simulink model "SPHERE_model"  (R2020a)
settings: Solver=ode4  StartTime=0.0  StopTime=20.0  FixedStep=0.01  RelTol=1e-3
values from neighbouring files (symbols this model uses):
  L = -[ M2*l*(-2*l + R) - 2*J2, 0, -2*M2*l*g ]    [Initial_script.m]    (also in Initial_script_test.m; Initial_script_test2.m)
  M = [ J1 + 2*J2 + M1*R^2 + M2*(2*l^2 - 3*R*l + R^2), -Tv, 2*l*g*M2 ]    [Initial_script.m]    (also in Initial_script_test.m; Initial_script_test2.m)
libraries: simulink x1
settings Model: Creator=Adrian  LastModifiedBy=Adrian

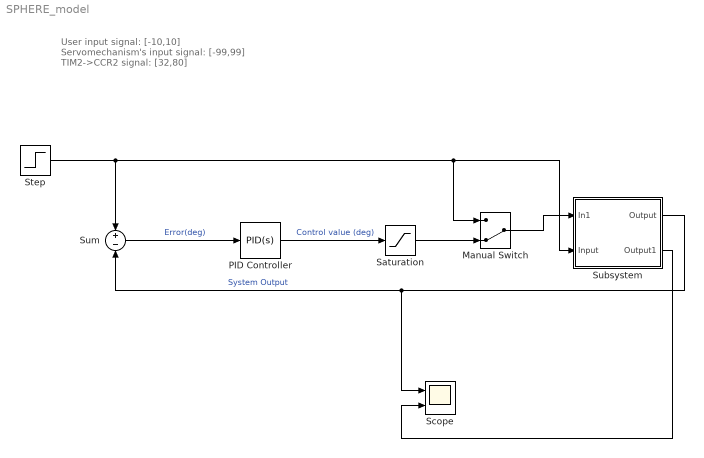
== system SPHERE_model ==
  note: User input signal: [-10,10]
      | Servomechanism's input signal: [-99,99]
      | TIM2->CCR2 signal: [32,80]
  Manual Switch : ManualSwitch  CurrentSetting=0
  PID Controller : simulink/Continuous/PID Controller  Controller=PID  Form=Parallel  TimeDomain=Continuous-time  UseExternalTs=off  SampleTime=-1  IntegratorMethod=Forward Euler  FilterMethod=Forward Euler  ControllerParametersSource=internal  P=1.5  I=0.2  D=0.1  UseFilter=on  N=100  TunerSelectOption=Transfer Function Based (PID Tuner App)  InitialConditionSource=internal  InitialConditionForIntegrator=0  InitialConditionForFilter=0  DifferentiatorICPrevScaledInput=0  ExternalReset=none  TrackingMode=off  Kt=1  LimitOutput=off  UpperSaturationLimit=inf  LowerSaturationLimit=-inf  LinearizeAsGain=on  AntiWindupMode=none  Kb=1  POutMin=[]  POutMax=[]  IOutMin=[]  IOutMax=[]  DOutMin=[]  DOutMax=[]  NOutMin=[]  NOutMax=[]  SumOutMin=[]  SumOutMax=[]  SaturationOutMin=[]  SaturationOutMax=[]  PParamMin=[]  PParamMax=[]  IParamMin=[]  IParamMax=[]  DParamMin=[]  DParamMax=[]  NParamMin=[]  NParamMax=[]  KbParamMin=[]  KbParamMax=[]  KtParamMin=[]  KtParamMax=[]  KbOutMin=[]  KbOutMax=[]  KtOutMin=[]  KtOutMax=[]  IntegratorOutMin=[]  IntegratorOutMax=[]  FilterOutMin=[]  FilterOutMax=[]  SumI1OutMin=[]  SumI1OutMax=[]  SumI2OutMin=[]  SumI2OutMax=[]  SumI3OutMin=[]  SumI3OutMax=[]  SumI4OutMin=[]  SumI4OutMax=[]  SumDOutMin=[]  SumDOutMax=[]  DifferentiatorOutMin=[]  DifferentiatorOutMax=[]  FilterDiffOutCoefMin=[]  FilterDiffOutCoefMax=[]  ReciprocalOutMin=[]  ReciprocalOutMax=[]  SumDenOutMin=[]  SumDenOutMax=[]  SumNumOutMin=[]  SumNumOutMax=[]  DivideOutMin=[]  DivideOutMax=[]  UdiffTsProdOutMin=[]  UdiffTsProdOutMax=[]  NTsProdOutMin=[]  NTsProdOutMax=[]  UintegralTsProdOutMin=[]  UintegralTsProdOutMax=[]  UngainTsProdOutMin=[]  UngainTsProdOutMax=[]  IntegratorContinuousStateAttributes=''  IntegratorStateMustResolveToSignalObject=off  IntegratorRTWStateStorageClass=Auto  FilterContinuousStateAttributes=''  FilterStateMustResolveToSignalObject=off  FilterRTWStateStorageClass=Auto  ParallelPVariant=InternalParameters  IdealPVariant=Disabled  IVariant=InternalParameters  DVariant=InternalParameters  IntegratorVariant=Continuous  SatVariant=Disabled  AWVariant=Passthrough  PCopyVariant=Disabled  TRVariant=Disabled  FdbkBlocksVariant=Forward  IdealPFdbkVariant=Disabled  SatFdbkVariant=Disabled  DerivativeFilterVariant=ContFilter  NVariant=InternalParameters  NCopyVariant=Disabled  FilterICVariant=InternalICsFilter  IntegratorICVariant=InternalICs  ExternalResetVariant=Disabled  TRSumVariant=Passthrough  SumFdbkVariant=Disabled  SumVariant=Sum_PID  TsampFilterVariant=InternalTs  TsampNgainVariant=Passthrough  TsampIntegralVariant=Passthrough
  Saturation : Saturate  UpperLimit=99  LowerLimit=-99
  Scope : Scope  NumInputPorts=2
  Step : Step  Time=3  After=15  SampleTime=0
  Subsystem : Subsystem
  Sum : Sum  Inputs=+|-
  wires:
  PID Controller/1 -> Saturation/1  "Control value (deg)"
  Saturation/1 -> Manual Switch/2
  Manual Switch/1 -> Subsystem/1(In1)
  Step/1 -> Subsystem/2(Input), Manual Switch/1, Sum/1
  Sum/1 -> PID Controller/1  "Error(deg)"
  Subsystem/1(Output) -> Scope/1, Sum/2  "System Output"
  Subsystem/2(Output1) -> Scope/2

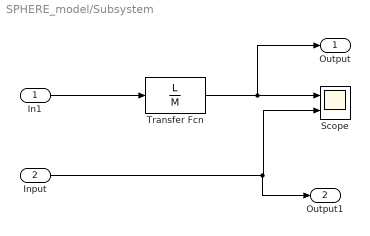
== system SPHERE_model/Subsystem ==
  In1 : Inport
  Input : Inport  Port=2
  Scope : Scope  NumInputPorts=2
  Transfer Fcn : TransferFcn  Numerator=L  Denominator=M
  Output : Outport
  Output1 : Outport  Port=2
  wires:
  In1/1 -> Transfer Fcn/1
  Transfer Fcn/1 -> Output/1, Scope/1
  Input/1 -> Output1/1, Scope/2
